simulink model "tres_sac15"  (R2014a)
settings: Solver=ode45  StartTime=0.0  StopTime=1  RelTol=1e-3
InitFcn:
  | clear functions
undefined symbols (not defined in the file or in its folder): OMNeT
libraries: tres_simulink_blockset x7
settings Model: ExtModeTrigMode=oneshot  ExtModeArmWhenConnect=off  ExtModeAutoUpdateStatusClock=off  Creator=anton  LastModifiedBy=matteo
settings DataIOCC: LimitDataPoints=off  SignalLoggingSaveFormat=ModelDataLogs
settings OptimizationCC: BlockReduction=off  BooleanDataType=off  InlineParams=on  ExpressionDepthLimit=2147483647
settings DebuggingCC: SaveWithParameterizedLinksMsg=none  UnderspecifiedInitializationDetection=Classic  SignalResolutionControl=TryResolveAllWithWarning  SolverPrmCheckMsg=none  MultiTaskDSMMsg=warning  MultiTaskCondExecSysMsg=none  FcnCallInpInsideContextMsg=UseLocalSettings  StateNameClashWarn=warning
settings HardwareCC: TargetUnknown=on
settings RTWCC: IncludeERTFirstTime=on
settings GRTTargetCC: CombineOutputUpdateFcns=off  GRTInterface=on

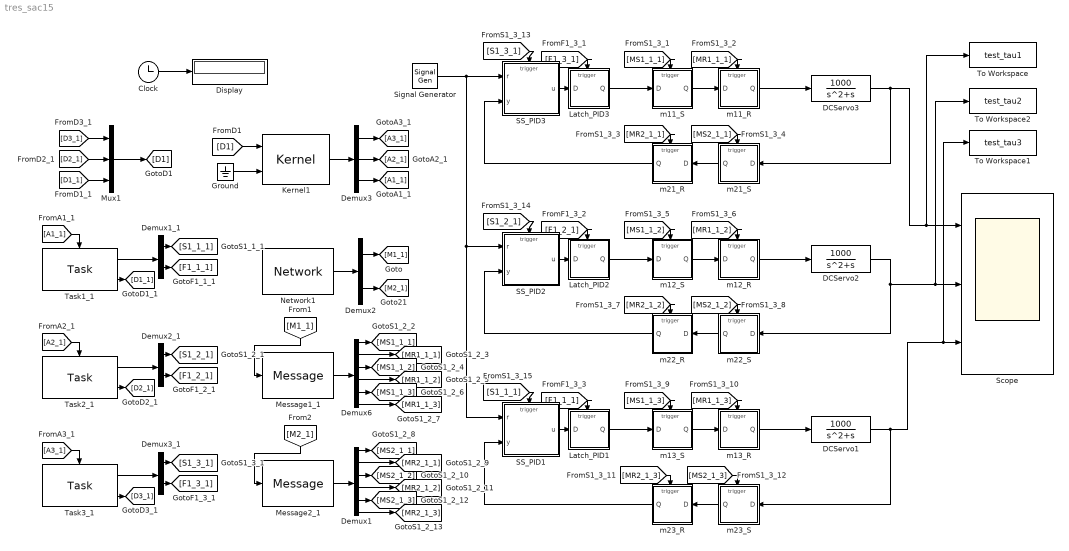
== system tres_sac15 ==
  Clock : Clock
  DCServo1 : TransferFcn  Numerator=[1000]  Denominator=[1 1 0]
  DCServo2 : TransferFcn  Numerator=[1000]  Denominator=[1 1 0]
  DCServo3 : TransferFcn  Numerator=[1000]  Denominator=[1 1 0]
  Demux1 : Demux  Outputs=6
  Demux1_1 : Demux  Outputs=2
  Demux2 : Demux  Outputs=2
  Demux2_1 : Demux  Outputs=2
  Demux3 : Demux  Outputs=3
  Demux3_1 : Demux  Outputs=2
  Demux6 : Demux  Outputs=6
  Display : Display
  Ground : Ground
  Kernel1 : tres_simulink_blockset/Kernel  taskset_descr_name=task_set_descr  scheduling_policy=DEADLINE_MONOTONIC  dead_miss_rule=Continue  time_res=Milli_Seconds  core_num=1  under_engine=RTSIM
  Latch_PID1 : Subsystem  TreatAsAtomicUnit=on
  Latch_PID2 : Subsystem  TreatAsAtomicUnit=on
  Latch_PID3 : Subsystem  TreatAsAtomicUnit=on
  Message1_1 : tres_simulink_blockset/Message  num_msg_objects=3
  Message2_1 : tres_simulink_blockset/Message  num_msg_objects=3
  Mux1 : Mux  Inputs=3
  Network1 : tres_simulink_blockset/Network  msgset_descr_name=msg_set_descr  time_res=Micro_Seconds  under_engine=OMNeT++  net_descr_name=ss_net_config  other_deps=[getenv('omnetpp_root'),'/inet/src/inet']
  SS_PID1 : Subsystem  TreatAsAtomicUnit=on
  SS_PID2 : Subsystem  TreatAsAtomicUnit=on
  SS_PID3 : Subsystem  TreatAsAtomicUnit=on
  Scope : Scope  NumInputPorts=3
      settings: YMin=-5~-5~-5  YMax=5~5~5
  Signal Generator : SignalGenerator  WaveForm=square  Frequency=1.5
  Task1_1 : tres_simulink_blockset/Task  conf_name=t1_descr
  Task2_1 : tres_simulink_blockset/Task  conf_name=t2_descr
  Task3_1 : tres_simulink_blockset/Task  conf_name=t3_descr
  To Workspace : ToWorkspace  VariableName=test_tau1  SaveFormat=Timeseries  SampleTime=-1
  To Workspace1 : ToWorkspace  VariableName=test_tau3  SaveFormat=Timeseries  SampleTime=-1
  To Workspace2 : ToWorkspace  VariableName=test_tau2  SaveFormat=Timeseries  SampleTime=-1
  m11_R : Subsystem  TreatAsAtomicUnit=on
  m11_S : Subsystem  TreatAsAtomicUnit=on
  m12_R : Subsystem  TreatAsAtomicUnit=on
  m12_S : Subsystem  TreatAsAtomicUnit=on
  m13_R : Subsystem  TreatAsAtomicUnit=on
  m13_S : Subsystem  TreatAsAtomicUnit=on
  m21_R : Subsystem  TreatAsAtomicUnit=on
  m21_S : Subsystem  TreatAsAtomicUnit=on
  m22_R : Subsystem  TreatAsAtomicUnit=on
  m22_S : Subsystem  TreatAsAtomicUnit=on
  m23_R : Subsystem  TreatAsAtomicUnit=on
  m23_S : Subsystem  TreatAsAtomicUnit=on
  wires:
  Clock/1 -> Display/1
  m11_S/1(Q) -> m11_R/1(D)
  m11_R/1(Q) -> DCServo3/1
  DCServo3/1 -> To Workspace/1, Scope/1, m21_S/1(D)
  [MS1_1_1] -> m11_S/Trigger
  [MR1_1_1] -> m11_R/Trigger
  [MR2_1_1] -> m21_R/Trigger
  [MS2_1_1] -> m21_S/Trigger
  m21_S/1(Q) -> m21_R/1(D)
  m21_R/1(Q) -> SS_PID3/2(y)
  Network1/1 -> Demux2/1
  Demux2/1 -> [M1_1]
  Demux2/2 -> [M2_1]
  Message1_1/1 -> Demux6/1
  Demux6/2 -> [MR1_1_1]
  Message2_1/1 -> Demux1/1
  [M2_1] -> Message2_1/1
  [M1_1] -> Message1_1/1
  DCServo2/1 -> m22_S/1(D), To Workspace2/1, Scope/2
  m12_S/1(Q) -> m12_R/1(D)
  m12_R/1(Q) -> DCServo2/1
  [MS1_1_2] -> m12_S/Trigger
  [MR1_1_2] -> m12_R/Trigger
  [MR2_1_2] -> m22_R/Trigger
  [MS2_1_2] -> m22_S/Trigger
  m22_S/1(Q) -> m22_R/1(D)
  m22_R/1(Q) -> SS_PID2/2(y)
  Signal Generator/1 -> SS_PID1/1(r), SS_PID2/1(r), SS_PID3/1(r)
  m13_S/1(Q) -> m13_R/1(D)
  m13_R/1(Q) -> DCServo1/1
  DCServo1/1 -> To Workspace1/1, Scope/3, m23_S/1(D)
  [MS1_1_3] -> m13_S/Trigger
  [MR1_1_3] -> m13_R/Trigger
  m23_S/1(Q) -> m23_R/1(D)
  m23_R/1(Q) -> SS_PID1/2(y)
  Kernel1/1 -> Demux3/1
  Demux3/1 -> [A3_1]
  Demux3/2 -> [A2_1]
  Demux3/3 -> [A1_1]
  [D1] -> Kernel1/1
  Ground/1 -> Kernel1/2
  Task1_1/2 -> [D1_1]
  [A1_1] -> Task1_1/Trigger
  Task1_1/1 -> Demux1_1/1
  Demux1_1/1 -> [S1_1_1]
  Demux1_1/2 -> [F1_1_1]
  Task2_1/2 -> [D2_1]
  [A2_1] -> Task2_1/Trigger
  Task2_1/1 -> Demux2_1/1
  Demux2_1/1 -> [S1_2_1]
  Demux2_1/2 -> [F1_2_1]
  Task3_1/2 -> [D3_1]
  [A3_1] -> Task3_1/Trigger
  Task3_1/1 -> Demux3_1/1
  Demux3_1/1 -> [S1_3_1]
  Demux3_1/2 -> [F1_3_1]
  [D3_1] -> Mux1/1
  [D2_1] -> Mux1/2
  [D1_1] -> Mux1/3
  Mux1/1 -> [D1]
  Demux6/1 -> [MS1_1_1]
  Demux6/3 -> [MS1_1_2]
  Demux6/4 -> [MR1_1_2]
  Demux6/5 -> [MS1_1_3]
  Demux6/6 -> [MR1_1_3]
  Demux1/2 -> [MR2_1_1]
  Demux1/1 -> [MS2_1_1]
  Demux1/3 -> [MS2_1_2]
  Demux1/4 -> [MR2_1_2]
  Demux1/5 -> [MS2_1_3]
  Demux1/6 -> [MR2_1_3]
  [MR2_1_3] -> m23_R/Trigger
  [MS2_1_3] -> m23_S/Trigger
  SS_PID3/1(u) -> Latch_PID3/1(D)
  Latch_PID3/1(Q) -> m11_S/1(D)
  [S1_3_1] -> SS_PID3/Trigger
  [F1_3_1] -> Latch_PID3/Trigger
  SS_PID2/1(u) -> Latch_PID2/1(D)
  Latch_PID2/1(Q) -> m12_S/1(D)
  [S1_2_1] -> SS_PID2/Trigger
  [F1_2_1] -> Latch_PID2/Trigger
  [S1_1_1] -> SS_PID1/Trigger
  [F1_1_1] -> Latch_PID1/Trigger
  SS_PID1/1(u) -> Latch_PID1/1(D)
  Latch_PID1/1(Q) -> m13_S/1(D)

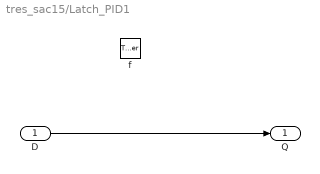
== system tres_sac15/Latch_PID1 ==
  D : Inport
  f : TriggerPort  TriggerType=function-call
  Q : Outport
  wires:
  D/1 -> Q/1

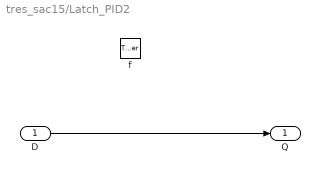
== system tres_sac15/Latch_PID2 ==
  D : Inport
  f : TriggerPort  TriggerType=function-call
  Q : Outport
  wires:
  D/1 -> Q/1

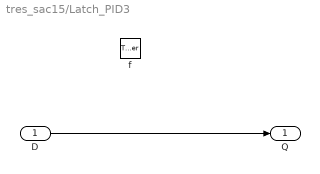
== system tres_sac15/Latch_PID3 ==
  D : Inport
  f : TriggerPort  TriggerType=function-call
  Q : Outport
  wires:
  D/1 -> Q/1

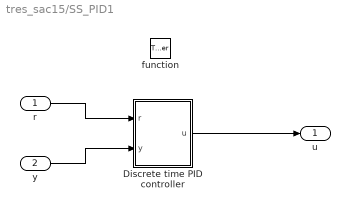
== system tres_sac15/SS_PID1 ==
  r : Inport
  y : Inport  Port=2
  function : TriggerPort  TriggerType=function-call
  Discrete time PID controller : Subsystem  mask{K=0.96, Ti=0.12, Td=0.049, beta=0.5, N=10, h=0.006}
  u : Outport
  wires:
  r/1 -> Discrete time PID controller/1(r)
  Discrete time PID controller/1(u) -> u/1
  y/1 -> Discrete time PID controller/2(y)

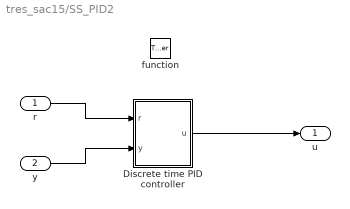
== system tres_sac15/SS_PID2 ==
  r : Inport
  y : Inport  Port=2
  function : TriggerPort  TriggerType=function-call
  Discrete time PID controller : Subsystem  mask{K=0.96, Ti=0.12, Td=0.049, beta=0.5, N=10, h=0.005}
  u : Outport
  wires:
  r/1 -> Discrete time PID controller/1(r)
  Discrete time PID controller/1(u) -> u/1
  y/1 -> Discrete time PID controller/2(y)

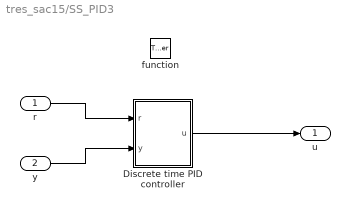
== system tres_sac15/SS_PID3 ==
  r : Inport
  y : Inport  Port=2
  function : TriggerPort  TriggerType=function-call
  Discrete time PID controller : Subsystem  mask{K=0.96, Ti=0.12, Td=0.049, beta=0.5, N=10, h=0.004}
  u : Outport
  wires:
  r/1 -> Discrete time PID controller/1(r)
  Discrete time PID controller/1(u) -> u/1
  y/1 -> Discrete time PID controller/2(y)

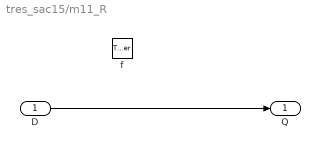
== system tres_sac15/m11_R ==
  D : Inport
  f : TriggerPort  TriggerType=function-call  PortDimensions=1
  Q : Outport
  wires:
  D/1 -> Q/1

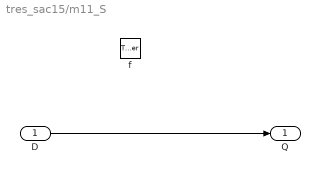
== system tres_sac15/m11_S ==
  D : Inport
  f : TriggerPort  TriggerType=function-call
  Q : Outport
  wires:
  D/1 -> Q/1

== system tres_sac15/m12_R ==
  D : Inport
  f : TriggerPort  TriggerType=function-call  PortDimensions=1
  Q : Outport
  wires:
  D/1 -> Q/1

== system tres_sac15/m12_S ==
  D : Inport
  f : TriggerPort  TriggerType=function-call
  Q : Outport
  wires:
  D/1 -> Q/1

== system tres_sac15/m13_R ==
  D : Inport
  f : TriggerPort  TriggerType=function-call  PortDimensions=1
  Q : Outport
  wires:
  D/1 -> Q/1

== system tres_sac15/m13_S ==
  D : Inport
  f : TriggerPort  TriggerType=function-call
  Q : Outport
  wires:
  D/1 -> Q/1

== system tres_sac15/m21_R ==
  D : Inport
  f : TriggerPort  TriggerType=function-call  PortDimensions=1
  Q : Outport
  wires:
  D/1 -> Q/1

== system tres_sac15/m21_S ==
  D : Inport
  f : TriggerPort  TriggerType=function-call
  Q : Outport
  wires:
  D/1 -> Q/1

== system tres_sac15/m22_R ==
  D : Inport
  f : TriggerPort  TriggerType=function-call  PortDimensions=1
  Q : Outport
  wires:
  D/1 -> Q/1

== system tres_sac15/m22_S ==
  D : Inport
  f : TriggerPort  TriggerType=function-call
  Q : Outport
  wires:
  D/1 -> Q/1

== system tres_sac15/m23_R ==
  D : Inport
  f : TriggerPort  TriggerType=function-call  PortDimensions=1
  Q : Outport
  wires:
  D/1 -> Q/1

== system tres_sac15/m23_S ==
  D : Inport
  f : TriggerPort  TriggerType=function-call
  Q : Outport
  wires:
  D/1 -> Q/1

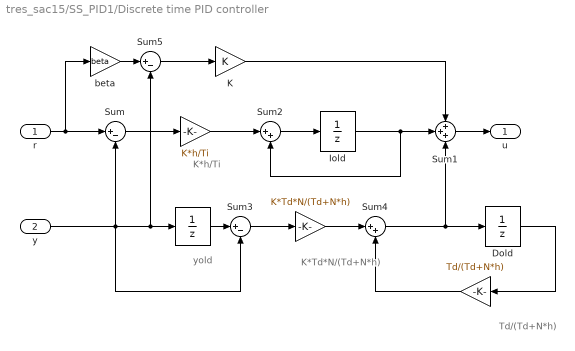
== system tres_sac15/SS_PID1/Discrete time PID controller ==
  note: K*h/Ti
  note: K*Td*N/(Td+N*h)
  note: Td/(Td+N*h)
  note: yold
  r : Inport
  y : Inport  Port=2
  " " : UnitDelay  SampleTime=-1
  " " : Gain  Gain=K*h/Ti  SaturateOnIntegerOverflow=on  OutDataTypeStr=Inherit: Same as input  ParamDataTypeStr=Inherit: Same as input
  "             " : Gain  Gain=K*Td*N/(Td+N*h)  SaturateOnIntegerOverflow=on  OutDataTypeStr=Inherit: Same as input  ParamDataTypeStr=Inherit: Same as input
  "              " : Gain  Gain=Td/(Td+N*h)  SaturateOnIntegerOverflow=on  OutDataTypeStr=Inherit: Same as input  ParamDataTypeStr=Inherit: Same as input
  Dold : UnitDelay  SampleTime=-1
  "Iold " : UnitDelay  SampleTime=-1
  K : Gain  Gain=K  SaturateOnIntegerOverflow=on  OutDataTypeStr=Inherit: Same as input  ParamDataTypeStr=Inherit: Same as input
  Sum : Sum  Inputs=|+-  SaturateOnIntegerOverflow=on  InputSameDT=on  OutDataTypeStr=Inherit: Same as first input
  Sum1 : Sum  Inputs=+++  SaturateOnIntegerOverflow=on  InputSameDT=on  OutDataTypeStr=Inherit: Same as first input
  Sum2 : Sum  Inputs=|++  SaturateOnIntegerOverflow=on  InputSameDT=on  OutDataTypeStr=Inherit: Same as first input
  Sum3 : Sum  Inputs=|+-  SaturateOnIntegerOverflow=on  InputSameDT=on  OutDataTypeStr=Inherit: Same as first input
  Sum4 : Sum  Inputs=|++  SaturateOnIntegerOverflow=on  InputSameDT=on  OutDataTypeStr=Inherit: Same as first input
  Sum5 : Sum  Inputs=|+-  SaturateOnIntegerOverflow=on  InputSameDT=on  OutDataTypeStr=Inherit: Same as first input
  beta : Gain  Gain=beta  SaturateOnIntegerOverflow=on  OutDataTypeStr=Inherit: Same as input  ParamDataTypeStr=Inherit: Same as input
  u : Outport
  wires:
  y/1 -> Sum/2, Sum3/2, " "/1, Sum5/2
  r/1 -> Sum/1, beta/1
  Sum1/1 -> u/1
  K/1 -> Sum1/1
  Sum2/1 -> "Iold "/1
  Dold/1 -> "              "/1
  "             "/1 -> Sum4/1
  Sum3/1 -> "             "/1
  Sum4/1 -> Dold/1, Sum1/3
  " "/1 -> Sum3/1
  "Iold "/1 -> Sum2/2, Sum1/2
  " "/1 -> Sum2/1
  Sum/1 -> " "/1
  "              "/1 -> Sum4/2
  beta/1 -> Sum5/1
  Sum5/1 -> K/1

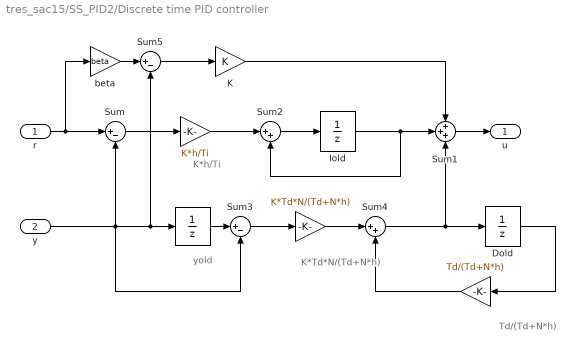
== system tres_sac15/SS_PID2/Discrete time PID controller ==
  note: K*h/Ti
  note: K*Td*N/(Td+N*h)
  note: Td/(Td+N*h)
  note: yold
  r : Inport
  y : Inport  Port=2
  " " : UnitDelay  SampleTime=-1
  " " : Gain  Gain=K*h/Ti  SaturateOnIntegerOverflow=on  OutDataTypeStr=Inherit: Same as input  ParamDataTypeStr=Inherit: Same as input
  "             " : Gain  Gain=K*Td*N/(Td+N*h)  SaturateOnIntegerOverflow=on  OutDataTypeStr=Inherit: Same as input  ParamDataTypeStr=Inherit: Same as input
  "              " : Gain  Gain=Td/(Td+N*h)  SaturateOnIntegerOverflow=on  OutDataTypeStr=Inherit: Same as input  ParamDataTypeStr=Inherit: Same as input
  Dold : UnitDelay  SampleTime=-1
  "Iold " : UnitDelay  SampleTime=-1
  K : Gain  Gain=K  SaturateOnIntegerOverflow=on  OutDataTypeStr=Inherit: Same as input  ParamDataTypeStr=Inherit: Same as input
  Sum : Sum  Inputs=|+-  SaturateOnIntegerOverflow=on  InputSameDT=on  OutDataTypeStr=Inherit: Same as first input
  Sum1 : Sum  Inputs=+++  SaturateOnIntegerOverflow=on  InputSameDT=on  OutDataTypeStr=Inherit: Same as first input
  Sum2 : Sum  Inputs=|++  SaturateOnIntegerOverflow=on  InputSameDT=on  OutDataTypeStr=Inherit: Same as first input
  Sum3 : Sum  Inputs=|+-  SaturateOnIntegerOverflow=on  InputSameDT=on  OutDataTypeStr=Inherit: Same as first input
  Sum4 : Sum  Inputs=|++  SaturateOnIntegerOverflow=on  InputSameDT=on  OutDataTypeStr=Inherit: Same as first input
  Sum5 : Sum  Inputs=|+-  SaturateOnIntegerOverflow=on  InputSameDT=on  OutDataTypeStr=Inherit: Same as first input
  beta : Gain  Gain=beta  SaturateOnIntegerOverflow=on  OutDataTypeStr=Inherit: Same as input  ParamDataTypeStr=Inherit: Same as input
  u : Outport
  wires:
  y/1 -> Sum/2, Sum3/2, " "/1, Sum5/2
  r/1 -> Sum/1, beta/1
  Sum1/1 -> u/1
  K/1 -> Sum1/1
  Sum2/1 -> "Iold "/1
  Dold/1 -> "              "/1
  "             "/1 -> Sum4/1
  Sum3/1 -> "             "/1
  Sum4/1 -> Dold/1, Sum1/3
  " "/1 -> Sum3/1
  "Iold "/1 -> Sum2/2, Sum1/2
  " "/1 -> Sum2/1
  Sum/1 -> " "/1
  "              "/1 -> Sum4/2
  beta/1 -> Sum5/1
  Sum5/1 -> K/1

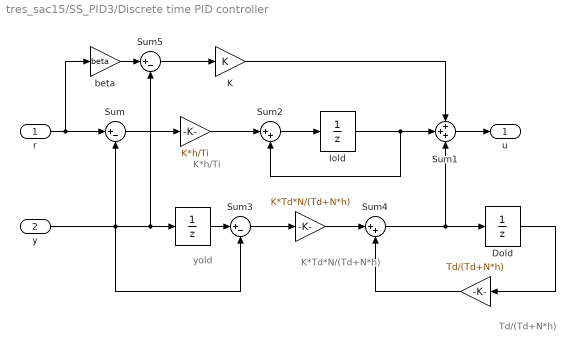
== system tres_sac15/SS_PID3/Discrete time PID controller ==
  note: K*h/Ti
  note: K*Td*N/(Td+N*h)
  note: Td/(Td+N*h)
  note: yold
  r : Inport
  y : Inport  Port=2
  " " : UnitDelay  SampleTime=-1
  " " : Gain  Gain=K*h/Ti  SaturateOnIntegerOverflow=on  OutDataTypeStr=Inherit: Same as input  ParamDataTypeStr=Inherit: Same as input
  "             " : Gain  Gain=K*Td*N/(Td+N*h)  SaturateOnIntegerOverflow=on  OutDataTypeStr=Inherit: Same as input  ParamDataTypeStr=Inherit: Same as input
  "              " : Gain  Gain=Td/(Td+N*h)  SaturateOnIntegerOverflow=on  OutDataTypeStr=Inherit: Same as input  ParamDataTypeStr=Inherit: Same as input
  Dold : UnitDelay  SampleTime=-1
  "Iold " : UnitDelay  SampleTime=-1
  K : Gain  Gain=K  SaturateOnIntegerOverflow=on  OutDataTypeStr=Inherit: Same as input  ParamDataTypeStr=Inherit: Same as input
  Sum : Sum  Inputs=|+-  SaturateOnIntegerOverflow=on  InputSameDT=on  OutDataTypeStr=Inherit: Same as first input
  Sum1 : Sum  Inputs=+++  SaturateOnIntegerOverflow=on  InputSameDT=on  OutDataTypeStr=Inherit: Same as first input
  Sum2 : Sum  Inputs=|++  SaturateOnIntegerOverflow=on  InputSameDT=on  OutDataTypeStr=Inherit: Same as first input
  Sum3 : Sum  Inputs=|+-  SaturateOnIntegerOverflow=on  InputSameDT=on  OutDataTypeStr=Inherit: Same as first input
  Sum4 : Sum  Inputs=|++  SaturateOnIntegerOverflow=on  InputSameDT=on  OutDataTypeStr=Inherit: Same as first input
  Sum5 : Sum  Inputs=|+-  SaturateOnIntegerOverflow=on  InputSameDT=on  OutDataTypeStr=Inherit: Same as first input
  beta : Gain  Gain=beta  SaturateOnIntegerOverflow=on  OutDataTypeStr=Inherit: Same as input  ParamDataTypeStr=Inherit: Same as input
  u : Outport
  wires:
  y/1 -> Sum/2, Sum3/2, " "/1, Sum5/2
  r/1 -> Sum/1, beta/1
  Sum1/1 -> u/1
  K/1 -> Sum1/1
  Sum2/1 -> "Iold "/1
  Dold/1 -> "              "/1
  "             "/1 -> Sum4/1
  Sum3/1 -> "             "/1
  Sum4/1 -> Dold/1, Sum1/3
  " "/1 -> Sum3/1
  "Iold "/1 -> Sum2/2, Sum1/2
  " "/1 -> Sum2/1
  Sum/1 -> " "/1
  "              "/1 -> Sum4/2
  beta/1 -> Sum5/1
  Sum5/1 -> K/1
